simulink model "task_5"  (R2019b)
settings: Solver=VariableStepAuto  StartTime=0.0  StopTime=100  RelTol=1e-3
PostLoadFcn:
  | % Path for this models parameters
  | modelPath = which(bdroot);  % Simulink model's path
  | [modelDirPath, name, ext] = fileparts(modelPath); % Get the path to model's parent directory
  | paramsPath = modelDirPath+"\params1.mat"; % Path to model parameters
  | 
  | % Load model parameters from file if the file exists, otherwise, use default values
  | if isfile(paramsPath)
  |     params = load(paramsPath).params;
  | else
  |     params = [1000; 25; 0.1];
  | end
  | 
  | % Speciying the initial condition for each state
  | x_0 = 0; % Initial distance (meters) from the reference point
  | v_0 = 20.12; % Initial velocity (m/s)
  | 
  | % Packing intial conditions into a vector
  | y_0 = [x_0; v_0];
PostSaveFcn:
  | % Path for this models parameters
  | modelPath = which(bdroot);  % Simulink model's path
  | [modelDirPath, name, ext] = fileparts(modelPath); % Get the path to model's parent directory
  | paramsPath = modelDirPath+"\params1.mat"; % Path to model parameters
  | 
  | % Save params to file
  | save(paramsPath, 'params');
settings Model: EnablePacing=on  PacingRate=20  Creator=Muhammad Saud  LastModifiedBy=Muhammad Saud

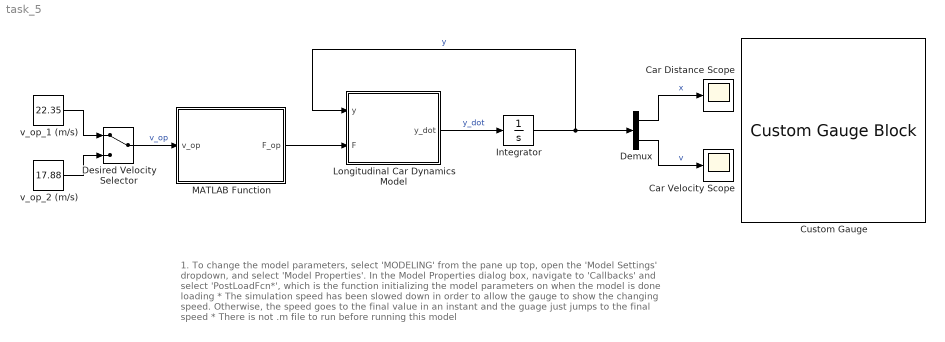
== system task_5 ==
  note: 1. To change the model parameters, select 'MODELING' from the pane up top, open the 'Model Settings' dropdown, and select 'Model Properties'. In the Model Properties dialog box, navigate to 'Callbacks' and select 'PostLoadFcn*', which is the function initializing the model parameters on when the model is done loading
      |
      | * The simulation speed has been slowed down in order to allow the gauge to show the changing speed. Otherwise, the speed goes to the final value in an instant and the guage just jumps to the final speed
      | * There is not .m file to run before running this model
  Car Distance Scope : Scope
  Car Velocity Scope : Scope
  Custom Gauge : CustomGaugeBlock  NeedleImage=data:image/svg+xml;base64,PD94bWwgdmVyc2lvbj0iMS4wIiBlbmNvZGluZz0idXRmLTgiPz4KPCEtLSBHZW5lcmF0b3I6IEFkb2JlIElsbHVzdHJhdG9yIDE5LjIuMSwgU1ZHIEV4cG9ydCBQbHVnLUluIC4gU1ZHIFZlcnNpb246IDYuMDAgQnVpbGQgMCkgIC0tPgo8c3ZnIHZlcnNpb249IjEuMSIgeG1sbnM9Imh0dHA6Ly93d3cudzMub3JnLzIwMDAvc3ZnIiB4bWxuczp4bGluaz0iaHR0cDovL3d3dy53My5vcmcvMTk5OS94bGluayIgeD0iMHB4IiB5PSIwcHgiCgkgdmlld0JveD0iMCAwIDIwMCA1MCIgc3R5bGU9ImVuYWJsZS1iYWNrZ3JvdW5kOm5ldyAw ...(+9940 chars)  NeedleXPos=0.38752017167580183  NeedleYPos=0.4823190446227708  NeedleHeight=0.10895934703145131  NeedleWidth=0.17950247846799225  NeedleInitialRotation=-59.94322499147643  BackgroundImage=data:image/svg+xml;base64,PD94bWwgdmVyc2lvbj0iMS4wIiBlbmNvZGluZz0iVVRGLTgiIHN0YW5kYWxvbmU9Im5vIj8+CjwhLS0gR2VuZXJhdG9yOiBBZG9iZSBJbGx1c3RyYXRvciAxOS4yLjEsIFNWRyBFeHBvcnQgUGx1Zy1JbiAuIFNWRyBWZXJzaW9uOiA2LjAwIEJ1aWxkIDApICAtLT4KCjxzdmcKICAgeG1sbnM6ZGM9Imh0dHA6Ly9wdXJsLm9yZy9kYy9lbGVtZW50cy8xLjEvIgogICB4bWxuczpjYz0iaHR0cDovL2NyZWF0aXZlY29tbW9ucy5vcmcvbnMjIgogICB4bWxuczpyZGY9Imh0dHA6Ly93d3cudzMub3JnLzE5OTkvMDIvMjItcmRmLXN5bnRh ...(+9660 chars)  GaugeMin=17  GaugeMax=27  GaugeArcDefined=true  GaugeArcRadius=0.12758687906784527  GaugeArcStrokeWidth=0.03731132857144653  GaugeArcRotation=240.5385250290321  GaugeArcRatio=0.8333333333333  GaugeArcTransparency=0  ValueArcColor=#1759b0  GaugeTickColor=#faf5c8  ScaleColorsJSON=[]  fixedAspectRatio=on  IsLinearGauge=false  GaugeTrackLeft=0.35  GaugeTrackTop=0.35  GaugeTrackHeight=0.1  GaugeTrackWidth=0.3  GaugeTrackRotation=0  ScaleMin=17
  Demux : Demux  Outputs=2
  Desired Velocity Selector : ManualSwitch
  Integrator : Integrator  InitialCondition=y_0
  Longitudinal Car Dynamics Model : MATLAB Function  TreatAsAtomicUnit=on
  MATLAB Function : MATLAB Function  TreatAsAtomicUnit=on
  v_op_1 (m/s) : Constant  Value=22.35
  v_op_2 (m/s) : Constant  Value=17.88
  wires:
  Longitudinal Car Dynamics Model/1(y_dot) -> Integrator/1  "y_dot"
  Integrator/1 -> Demux/1, Longitudinal Car Dynamics Model/1(y)  "y"
  Demux/2 -> Car Velocity Scope/1  "v"
  Demux/1 -> Car Distance Scope/1  "x"
  v_op_1 (m/s)/1 -> Desired Velocity Selector/1
  v_op_2 (m/s)/1 -> Desired Velocity Selector/2
  Desired Velocity Selector/1 -> MATLAB Function/1(v_op)  "v_op"
  MATLAB Function/1(F_op) -> Longitudinal Car Dynamics Model/2(F)

== matlab function task_5/MATLAB Function ==
  data: v_op input; F_op output; params parameter
function F_op = feedforward_map(v_op, params)
    %% Specifies mapping from nominal velocity to nominal force
    % Inputs:
    % -------
    % v_op: The nominal velocity (velocity at equilibrium point)
    % params: A vector of system parameters
    %         It is a 3-dimensional column vector of the form:
    %         [mass; ground_friction-coefficient; drag_coefficient]
    %
    % Output:
    % -------
    % F_op: The nominal force (force at equilibrium point)
    
    % Unpacking Parameters
    m = params(1);
    b = params(2);
    cd = params(3);
    
    % Defining feedforward mapping from v_0 to F_0
    F_op = b*v_op + cd*v_op^2;

end % end feedforward_map function

== matlab function task_5/Longitudinal Car Dynamics Model ==
  data: y input; y_dot output; F input; params parameter
function y_dot = car(y, F, params)
    %% This subroutine defines the longitudal car dynamics
    % Inputs
    % ------
    % y: State vector
    %    It is a 2-dimensional column vector of the form:
    %    [distance; car_velocity]
    % F: Input force (acting on the car)
    % params: A vector of model parameters
    %         It is a 3-dimensional column vector of the form:
    %         [mass; ground_friction-coefficient; drag_coefficient]
    %
    % Outputs
    % -------
    % y_dot: Time derivative of the state vector
    %        It has the same dimension as the state vector (y) and is of
    %        the form:
    %        [car_velocity; acceleration];
    
    % Unpacking parameters
    m = params(1);
    b = params(2);
    cd = params(3);
    
    % Defining the ODEs describing system's dynamics
    y_dot1 = y(2); % ODE defining car velocity
    y_dot2 = (F-b*y(2)-cd*y(2)^2)/m; % ODE defining car acceleration
    
    % Pack the differentiated states into a vector
    y_dot = [y_dot1; y_dot2];
    
end % end car subroutine
